simulink model "v2021_10_27_Modello_SITL_AENEA_2020b"  (R2020b)
settings: Solver=ode4  StartTime=0.0  StopTime=0.01  FixedStep=0.01  RelTol=1e-3
values from neighbouring files (symbols this model uses):
  alphavec_rad = deg2rad(alphavec)    [v2021_10_27_calcoloAerodinamica.m]
  attuatore_Amax = 20*(pi/180)    (= 0.349065850399)    [v2021_10_27_avvioSITL.m]    (also in v2021_10_27_calcoloAerodinamica.m)
  attuatore_Emax = 25*(pi/180)    (= 0.436332312999)    [v2021_10_27_avvioSITL.m]    (also in v2021_10_27_calcoloAerodinamica.m)
  attuatore_Rmax = 25*(pi/180)    (= 0.436332312999)    [v2021_10_27_avvioSITL.m]    (also in v2021_10_27_calcoloAerodinamica.m)
  b = 2.62    [v2021_10_27_calcoloAerodinamica.m]
  betavec_rad = deg2rad(betavec)    [v2021_10_27_calcoloAerodinamica.m]
  c = .32    (= 0.32)    [v2021_10_27_calcoloAerodinamica.m]
  cbar = .32    (= 0.32)    [v2021_10_27_calcoloAerodinamica.m]
  CD0 = 0.024    [v2021_10_27_calcoloAerodinamica.m]
  Clp = -0.5058    [v2021_10_27_calcoloAerodinamica.m]
  CLq = 19.166    [v2021_10_27_calcoloAerodinamica.m]
  Clr = 0.1459    [v2021_10_27_calcoloAerodinamica.m]
  Cmq = -81.796    [v2021_10_27_calcoloAerodinamica.m]
  Cnp = 0.007507    [v2021_10_27_calcoloAerodinamica.m]
  Cnr = -1.2593    [v2021_10_27_calcoloAerodinamica.m]
  CYp = 0.050728    [v2021_10_27_calcoloAerodinamica.m]
  CYr = 0.358925    [v2021_10_27_calcoloAerodinamica.m]
  deltaAtrim = 0    [v2021_10_27_avvioSITL.m]
  deltaEtrim = 0    [v2021_10_27_avvioSITL.m]
  deltaRtrim = 0    [v2021_10_27_avvioSITL.m]
  deltaTtrim = 0.1    [v2021_10_27_avvioSITL.m]
  Dprop = 2*Rprop    (= 0.5334)    [v2021_10_27_calcoloAerodinamica.m]
  g = [0 0 9.81]'    [v2021_10_27_calcoloAerodinamica.m]
  HINI = -State0.Pos0(3)    [v2021_10_27_avvioSITL.m]
  Jeng = 0    [v2021_10_27_calcoloAerodinamica.m]
  Jprop = mprop*(Dprop^2)/12    (= 0.00422031414)    [v2021_10_27_calcoloAerodinamica.m]
  latitudineINI = 41.854432*pi/180    (= 0.730497644952)    [v2021_10_27_avvioSITL.m]
  longitudineINI = 12.306650*pi/180    (= 0.214791562391)    [v2021_10_27_avvioSITL.m]
  matricepolinomi = [0.0816560564319 0.0869820125665 0.0279748858868 -4.51852057237 0.0146653626785 -0.925775006168 8.18052218957e-06 -1.47322908992e-05 7.59644694438e-06 0.00246695371279 9.02269223066e-06 0.000559334242525 ... (126 elements, 6x21)]    [coefficienti_curve_renard.mat]
  PWM_Aileron = rad2deg(deltaAtrim)*9+1503    [v2021_10_27_avvioSITL.m]
  PWM_Elevator = rad2deg(deltaEtrim)*(447/50)+(3007/2)    [v2021_10_27_avvioSITL.m]
  PWM_Rudder = rad2deg(deltaRtrim)*(447/50)+(3007/2)    [v2021_10_27_avvioSITL.m]
  PWM_Throttle = (deltaTtrim)*800+1100    (= 1180)    [v2021_10_27_avvioSITL.m]
  q = stato(11)    [measure_F1B.m]
  r = stato(12)    [measure_F1B.m]
  rACtG = rACtP-rGP    [v2021_10_27_calcoloAerodinamica.m]
  rACwG = rACwP-rGP    [v2021_10_27_calcoloAerodinamica.m]
  rAHRSG = rAHRSP-rGP    [v2021_10_27_calcoloAerodinamica.m]
  rho = 1.21330    (= 1.2133)    [v2021_10_27_calcoloAerodinamica.m]
  rLEG = rLEP-rGP    [v2021_10_27_calcoloAerodinamica.m]
  rmglG = rmglP-rGP    [v2021_10_27_calcoloAerodinamica.m]
  rmgrG = rmgrP-rGP    [v2021_10_27_calcoloAerodinamica.m]
  rngG = rngP-rGP    [v2021_10_27_calcoloAerodinamica.m]
  rNPG = rNPP-rGP    [v2021_10_27_calcoloAerodinamica.m]
  rPG = -rGP    [v2021_10_27_calcoloAerodinamica.m]
  Rprop = 0.2667    [v2021_10_27_calcoloAerodinamica.m]
  S = b*cbar    (= 0.8384)    [v2021_10_27_calcoloAerodinamica.m]
  sensori_FreqCampionamento_pitot = 0.02    [v2021_10_27_avvioSITL.m]
  sensori_RumoreSampleTime = 0.02    [v2021_10_27_avvioSITL.m]
  sensori_varianza = 0.0000    (= 0)    [v2021_10_27_avvioSITL.m]
  tsamp = 0.02    [v2021_10_27_avvioSITL.m]
  V_cruise = input('inserire un valore desiderato per V_cruise: ')    [trimCalc.m]    (also in v2021_10_27_trimCalc.m = input('inserire un valore desiderato per V_cruise [m/s]: '))
  W = m*g    [v2021_10_27_calcoloAerodinamica.m]
  WP_AL = [     0 20 0 0 41.807822 12.589274 3 ... (first row only)    [v2021_10_27_avvioSITL.m]
  WP_db_info = [0 0 0 0 1 3;              0 0 0 0 2 3;              0 0 0 0 3 3;              0 0 0 0 0 0]    [v2021_10_27_avvioSITL.m]
  WP_db_param = [ ... (first row only)    [v2021_10_27_avvioSITL.m]
  Zeng = rPG(3)    [v2021_10_27_calcoloAerodinamica.m]
  Zpista = 0    [v2021_10_27_avvioSITL.m]
undefined symbols (not defined in the file or in its folder): beta_phi, beta_psi, beta_theta, CldA, CLdE, CldR, CmdE, CndA, CndR, CYdA, CYdR, delay_ahrs, delay_bmp, delay_gps, Earth, F, h_home, J_vec, mean_ax, mean_ay, mean_az, mean_p, mean_q, mean_r, MIL, P_ref, Receive, seed_ahrs, seed_baro, seed_gps, Send, State0, Std_con_lat, Std_con_long, Std_vel, T0_ref, Ta_lat, Ta_long, Ts_ahrs, Ts_bmp, Ts_gps, Var_heading_static, Var_V_hor_static, WGS84, White_ax, White_ay, White_az, White_gm_phi, White_gm_psi, White_gm_theta, White_p, White_pressione, White_r
libraries: simulink_extras x27, aerolibfltsims x5, aerolibwind2 x3, aerolibasang x2, simulink x2, shared6dof x1, pid_lib x1, aerolibatmos2 x1, aerolibanimutils x1
(part 2 of 3)

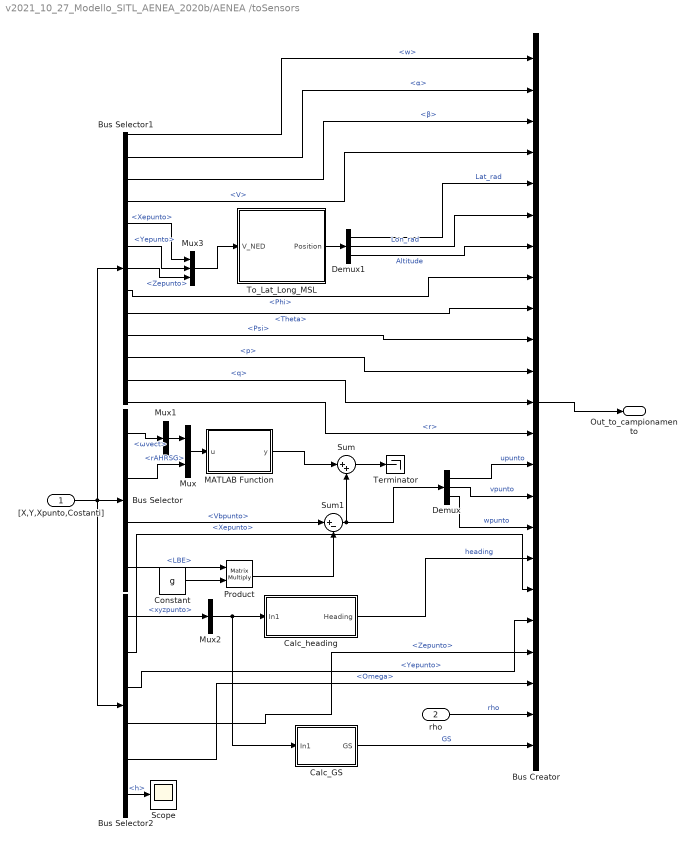
== system v2021_10_27_Modello_SITL_AENEA_2020b/AENEA /toSensors ==
  "[X,Y,Xpunto,Costanti]" : Inport
  rho : Inport  Port=2
  Bus Creator : BusCreator  Inputs=23
  Bus Selector : BusSelector  OutputSignals=X.ωvect,Costanti.Vett_caratteristici.rAHRSG,Xpunto.Vbpunto,Y.LBE
  Bus Selector1 : BusSelector  OutputSignals=X.uvw.w,Y.Vbpolare.α,Y.Vbpolare.β,Y.Vbpolare.V,Xpunto.xyzpunto.Xepunto,Xpunto.xyzpunto.Yepunto,Xpunto.xyzpunto.Zepunto,X.PhiThetaPsi.Phi,X.PhiThetaPsi.Theta,X.PhiThetaPsi.Psi,X.ωvect.p,X.ωvect.q,X.ωvect.r
  Bus Selector2 : BusSelector  OutputSignals=Xpunto.xyzpunto,Xpunto.xyzpunto.Xepunto,Xpunto.xyzpunto.Yepunto,Xpunto.xyzpunto.Zepunto,Y.Omega,X.xyz.h
  Calc_GS : Subsystem
  Calc_heading : Subsystem
  Constant : Constant  Value=g
  Demux : Demux  Outputs=3
  Demux1 : Demux  Outputs=3
  MATLAB Function : MATLAB Function  TreatAsAtomicUnit=on
  Mux : Mux  Inputs=2
  Mux1 : Mux  Inputs=1
  Mux2 : Mux  Inputs=1
  Mux3 : Mux  Inputs=3
  Product : Product  Multiplication=Matrix(*)
  Scope : Scope
  Sum : Sum  Inputs=|++
  Sum1 : Sum  Inputs=|+-
  Terminator : Terminator
  To_Lat_Long_MSL : Subsystem
  Out_to_campionamento : Outport  VectorParamsAs1DForOutWhenUnconnected=off
  wires:
  "[X,Y,Xpunto,Costanti]"/1 -> Bus Selector2/1, Bus Selector1/1, Bus Selector/1
  Mux/1 -> MATLAB Function/1(u)
  Mux1/1 -> Mux/1
  Bus Selector/4 -> Product/1  "<LBE>"
  Constant/1 -> Product/2
  Mux2/1 -> Calc_GS/1(In1), Calc_heading/1(In1)
  Bus Selector2/1 -> Mux2/1  "<xyzpunto>"
  Bus Selector1/1 -> Bus Creator/1  "<w>"
  Bus Selector1/2 -> Bus Creator/2  "<α>"
  Bus Selector1/3 -> Bus Creator/3  "<β>"
  Bus Creator/1 -> Out_to_campionamento/1
  Bus Selector1/4 -> Bus Creator/4  "<V>"
  Bus Selector1/8 -> Bus Creator/8  "<Phi>"
  Bus Selector1/9 -> Bus Creator/9  "<Theta>"
  Bus Selector1/10 -> Bus Creator/10  "<Psi>"
  Bus Selector1/11 -> Bus Creator/11  "<p>"
  Bus Selector1/12 -> Bus Creator/12  "<q>"
  Bus Selector1/13 -> Bus Creator/13  "<r>"
  Demux/1 -> Bus Creator/14  "upunto"
  Demux/2 -> Bus Creator/15  "vpunto"
  Demux/3 -> Bus Creator/16  "wpunto"
  Calc_heading/1(Heading) -> Bus Creator/17  "heading"
  Bus Selector2/5 -> Bus Creator/21  "<Omega>"
  rho/1 -> Bus Creator/22  "rho"
  Calc_GS/1(GS) -> Bus Creator/23  "GS"
  Mux3/1 -> To_Lat_Long_MSL/1(V_NED)
  Bus Selector1/7 -> Mux3/3  "<Zepunto>"
  Bus Selector1/6 -> Mux3/2  "<Yepunto>"
  Bus Selector1/5 -> Mux3/1  "<Xepunto>"
  To_Lat_Long_MSL/1(Position) -> Demux1/1
  Demux1/1 -> Bus Creator/5  "Lat_rad"
  Demux1/2 -> Bus Creator/6  "Lon_rad"
  Demux1/3 -> Bus Creator/7  "Altitude"
  Bus Selector2/2 -> Bus Creator/18  "<Xepunto>"
  Bus Selector2/3 -> Bus Creator/19  "<Yepunto>"
  Bus Selector2/4 -> Bus Creator/20  "<Zepunto>"
  Bus Selector/1 -> Mux1/1  "<ωvect>"
  Bus Selector/2 -> Mux/2  "<rAHRSG>"
  MATLAB Function/1(y) -> Sum/1
  Sum/1 -> Terminator/1
  Product/1 -> Sum1/2
  Bus Selector2/6 -> Scope/1  "<h>"
  Sum1/1 -> Demux/1, Sum/2
  Bus Selector/3 -> Sum1/1  "<Vbpunto>"

== system v2021_10_27_Modello_SITL_AENEA_2020b/Ricezione segnali2/Subsystem1 ==
  In1 : Inport
  In2 : Inport  Port=2
  In3 : Inport  Port=3
  In4 : Inport  Port=4
  AILERON : Subsystem
  Degrees to Radians : simulink_extras/Transformations/Degrees to Radians
  Degrees to Radians1 : simulink_extras/Transformations/Degrees to Radians
  Degrees to Radians2 : simulink_extras/Transformations/Degrees to Radians
  ELEVATOR : Subsystem
  RUDDER : Subsystem
  Scope : Scope  NumInputPorts=2
  Scope1 : Scope
  Scope2 : Scope  NumInputPorts=2
  Scope3 : Scope
  Scope4 : Scope
  THROTTLE : Subsystem
  Out1 : Outport  VectorParamsAs1DForOutWhenUnconnected=off
  Out2 : Outport  Port=2  VectorParamsAs1DForOutWhenUnconnected=off
  Out3 : Outport  Port=3  VectorParamsAs1DForOutWhenUnconnected=off
  Out4 : Outport  Port=4  VectorParamsAs1DForOutWhenUnconnected=off
  wires:
  In3/1 -> AILERON/1(In1)
  In4/1 -> RUDDER/1(In1)
  In2/1 -> Scope/1, ELEVATOR/1(In1)
  In1/1 -> Scope2/1, THROTTLE/1(In1)
  Degrees to Radians2/1 -> Out4/1, Scope4/1  "Timone"
  Degrees to Radians1/1 -> Out3/1, Scope3/1  "Alettoni"
  Degrees to Radians/1 -> Scope/2, Scope1/1, Out2/1  "Equilibratore"
  THROTTLE/1(Out1) -> Scope2/2, Out1/1  "Manetta"
  ELEVATOR/1(Out1) -> Degrees to Radians/1  "Equilibratore"
  AILERON/1(Out1) -> Degrees to Radians1/1  "Alettoni"
  RUDDER/1(Out1) -> Degrees to Radians2/1  "Timone"

== system v2021_10_27_Modello_SITL_AENEA_2020b/ 1/GPS1/Subsystem ==
  Lat : Inport
  C/Lat1 : Constant  Value=Std_con_lat
  Delay_gps : TransportDelay  DelayTime=delay_gps  InitialOutput=latitudineINI
  Gain : Gain  Gain=1/Ta_lat  SaturateOnIntegerOverflow=on  OutDataTypeStr=Inherit: Same as input  ParamDataTypeStr=Inherit: Same as input
  Integrator : Integrator
  Multiply : Product
  Multiply1 : Product
  Sum : Sum  Inputs=|+-  InputSameDT=on  SaturateOnIntegerOverflow=on  OutDataTypeStr=Inherit: Same as first input
  Sum1 : Sum  Inputs=|++  InputSameDT=on  SaturateOnIntegerOverflow=on  OutDataTypeStr=Inherit: Same as first input
  To Workspace : ToWorkspace  Commented=on  VariableName=errore_lat  SaveFormat=Timeseries  SampleTime=-1
  White Noise : RandomNumber  Seed=seed_gps  SampleTime=Ts_gps
  Out1 : Outport  VectorParamsAs1DForOutWhenUnconnected=off
  wires:
  Sum1/1 -> Out1/1
  Integrator/1 -> Gain/1, Sum1/2, To Workspace/1
  Sum/1 -> Integrator/1
  Delay_gps/1 -> Multiply1/1, Sum1/1
  Gain/1 -> Sum/2
  White Noise/1 -> Multiply/2
  Multiply/1 -> Sum/1
  Lat/1 -> Delay_gps/1
  C/Lat1/1 -> Multiply1/2
  Multiply1/1 -> Multiply/1

== system v2021_10_27_Modello_SITL_AENEA_2020b/ 1/GPS1/Subsystem1 ==
  Long : Inport
  C/Long1 : Constant  Value=Std_con_long
  Delay_gps : TransportDelay  DelayTime=delay_gps  InitialOutput=longitudineINI
  Gain1 : Gain  Gain=1/Ta_long  SaturateOnIntegerOverflow=on  OutDataTypeStr=Inherit: Same as input  ParamDataTypeStr=Inherit: Same as input
  Integrator : Integrator
  Multiply : Product
  Multiply1 : Product
  Sum : Sum  Inputs=|+-  InputSameDT=on  SaturateOnIntegerOverflow=on  OutDataTypeStr=Inherit: Same as first input
  Sum1 : Sum  Inputs=|++  InputSameDT=on  SaturateOnIntegerOverflow=on  OutDataTypeStr=Inherit: Same as first input
  To Workspace : ToWorkspace  VariableName=errore_long  SaveFormat=Timeseries  SampleTime=-1
  White Noise : RandomNumber  Seed=seed_gps  SampleTime=Ts_gps
  long_out : Outport  VectorParamsAs1DForOutWhenUnconnected=off
  wires:
  Multiply/1 -> Sum/1
  White Noise/1 -> Multiply/2
  Gain1/1 -> Sum/2
  Sum1/1 -> long_out/1
  Delay_gps/1 -> Multiply1/1, Sum1/1
  Sum/1 -> Integrator/1
  Integrator/1 -> Sum1/2, To Workspace/1, Gain1/1
  Multiply1/1 -> Multiply/1
  C/Long1/1 -> Multiply1/2
  Long/1 -> Delay_gps/1

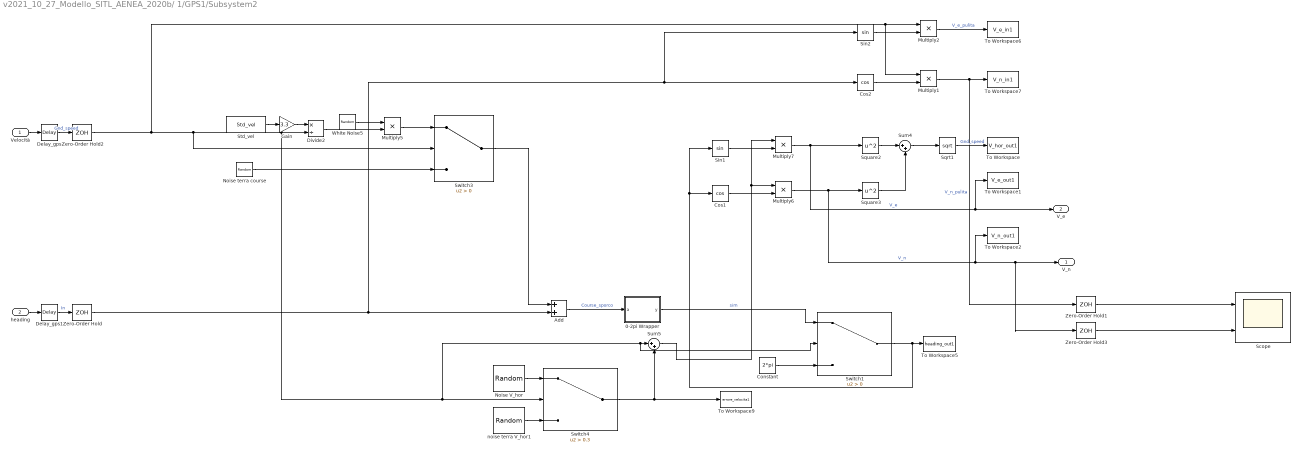
== system v2021_10_27_Modello_SITL_AENEA_2020b/ 1/GPS1/Subsystem2 ==
  Velocità : Inport
  heading : Inport  Port=2
  0-2pi Wrapper : MATLAB Function  TreatAsAtomicUnit=on
  Add : Sum
  Constant : Constant  Value=2*pi
  Cos1 : Trigonometry  Operator=cos
  Cos2 : Trigonometry  Operator=cos
  Delay_gps : TransportDelay  DelayTime=delay_gps  InitialOutput=V_cruise
  Delay_gps1 : TransportDelay  DelayTime=delay_gps
  Divide2 : Product  Inputs=*/
  Gain : Gain  Gain=3.3
  Multiply{1..2,5..7} (5 alike) : Product
  Noise V_hor : RandomNumber  Variance=Std_vel^2  Seed=seed_gps  SampleTime=Ts_gps
  Noise terra course : RandomNumber  Variance=Var_heading_static  Seed=seed_gps  SampleTime=0.02
  Scope : Scope  NumInputPorts=2
  Sin1 : Trigonometry
  Sin2 : Trigonometry
  Sqrt1 : Sqrt  SaturateOnIntegerOverflow=on
  Square2 : Math  Operator=square  SignedPower=on  SaturateOnIntegerOverflow=on
  Square3 : Math  Operator=square  SignedPower=on  SaturateOnIntegerOverflow=on
  Std_vel : Constant  Value=Std_vel
  Sum4 : Sum  Inputs=|++
  Sum5 : Sum  Inputs=|++
  Switch1 : Switch  Criteria=u2 > Threshold
  Switch3 : Switch  Criteria=u2 > Threshold
  Switch4 : Switch  Criteria=u2 > Threshold  Threshold=0.3
  To Workspace : ToWorkspace  VariableName=V_hor_out1  SaveFormat=Timeseries  SampleTime=-1
  To Workspace1 : ToWorkspace  VariableName=V_e_out1  SaveFormat=Timeseries  SampleTime=-1
  To Workspace2 : ToWorkspace  VariableName=V_n_out1  SaveFormat=Timeseries  SampleTime=-1
  To Workspace5 : ToWorkspace  VariableName=heading_out1  SaveFormat=Timeseries  SampleTime=-1
  To Workspace6 : ToWorkspace  VariableName=V_e_in1  SaveFormat=Timeseries  SampleTime=-1
  To Workspace7 : ToWorkspace  VariableName=V_n_in1  SaveFormat=Timeseries  SampleTime=-1
  To Workspace9 : ToWorkspace  VariableName=errore_velocita1  SaveFormat=Timeseries  SampleTime=-1
  White Noise5 : RandomNumber  Variance=0.1  Seed=seed_gps  SampleTime=0.02
  Zero-Order Hold : ZeroOrderHold  SampleTime=0.02
  Zero-Order Hold1 : ZeroOrderHold  SampleTime=0.2
  Zero-Order Hold2 : ZeroOrderHold  SampleTime=0.02
  Zero-Order Hold3 : ZeroOrderHold  SampleTime=0.2
  noise terra V_hor1 : RandomNumber  Variance=Var_V_hor_static  Seed=seed_gps  SampleTime=Ts_gps
  "V_n " : Outport  VectorParamsAs1DForOutWhenUnconnected=off
  V_e : Outport  Port=2  VectorParamsAs1DForOutWhenUnconnected=off
  wires:
  Zero-Order Hold2/1 -> Multiply2/1, Multiply1/1, Switch3/2, Divide2/2, Switch4/2, Sum5/1, Switch1/2
  Zero-Order Hold/1 -> Add/2, Sin2/1, Cos2/1
  Switch1/1 -> To Workspace5/1, Cos1/1, Sin1/1
  Constant/1 -> Switch1/3
  Sqrt1/1 -> To Workspace/1  "Gnd_speed"
  Divide2/1 -> Multiply5/2
  Velocità/1 -> Delay_gps/1
  heading/1 -> Delay_gps1/1
  Sin2/1 -> Multiply2/2
  Sin1/1 -> Multiply7/2
  Noise terra course/1 -> Switch3/3
  0-2pi Wrapper/1(y) -> Switch1/1  "sim"
  Cos2/1 -> Multiply1/2
  Multiply2/1 -> To Workspace6/1  "V_e_pulita"
  Multiply1/1 -> Zero-Order Hold1/1, To Workspace7/1  "V_n_pulita"
  Noise V_hor/1 -> Switch4/1
  Switch3/1 -> Add/1
  Cos1/1 -> Multiply6/2
  Sum4/1 -> Sqrt1/1
  Multiply7/1 -> Square2/1, V_e/1, To Workspace1/1  "V_e"
  White Noise5/1 -> Multiply5/1
  Delay_gps/1 -> Zero-Order Hold2/1  "Gnd_speed"
  Sum5/1 -> Multiply7/1, Multiply6/1
  Multiply6/1 -> Square3/1, To Workspace2/1, Zero-Order Hold3/1, "V_n "/1  "V_n"
  Square2/1 -> Sum4/1
  Multiply5/1 -> Switch3/1
  Add/1 -> 0-2pi Wrapper/1(a)  "Course_sporco"
  Delay_gps1/1 -> Zero-Order Hold/1  "In"
  Square3/1 -> Sum4/2
  noise terra V_hor1/1 -> Switch4/3
  Switch4/1 -> Sum5/2, To Workspace9/1
  Zero-Order Hold1/1 -> Scope/1
  Zero-Order Hold3/1 -> Scope/2
  Std_vel/1 -> Gain/1
  Gain/1 -> Divide2/1

== system v2021_10_27_Modello_SITL_AENEA_2020b/ 1/int1/INT16  ==
  <u> : Inport
  Data Type Conversion : DataTypeConversion  OutDataTypeStr=int16  LockScale=on
  Data Type Conversion1 : DataTypeConversion  OutDataTypeStr=double  LockScale=on
  Gain : Gain  Gain=100
  Gain1 : Gain  Gain=1/100
  Out1 : Outport  VectorParamsAs1DForOutWhenUnconnected=off
  wires:
  <u>/1 -> Gain/1
  Gain1/1 -> Out1/1
  Gain/1 -> Data Type Conversion/1
  Data Type Conversion/1 -> Data Type Conversion1/1
  Data Type Conversion1/1 -> Gain1/1

== system v2021_10_27_Modello_SITL_AENEA_2020b/ 1/int16/INT16  ==
  <u> : Inport
  Data Type Conversion : DataTypeConversion  OutDataTypeStr=int16  LockScale=on
  Data Type Conversion1 : DataTypeConversion  OutDataTypeStr=double  LockScale=on
  Gain : Gain  Gain=100
  Gain1 : Gain  Gain=1/100
  Out1 : Outport  VectorParamsAs1DForOutWhenUnconnected=off
  wires:
  Data Type Conversion1/1 -> Gain1/1
  Data Type Conversion/1 -> Data Type Conversion1/1
  Gain/1 -> Data Type Conversion/1
  Gain1/1 -> Out1/1
  <u>/1 -> Gain/1

== system v2021_10_27_Modello_SITL_AENEA_2020b/ 1/int16_rad /INT16  ==
  <u> : Inport
  Data Type Conversion : DataTypeConversion  OutDataTypeStr=int16  LockScale=on
  Data Type Conversion1 : DataTypeConversion  OutDataTypeStr=double  LockScale=on
  Gain : Gain  Gain=100
  Gain1 : Gain  Gain=1/100
  Out1 : Outport  VectorParamsAs1DForOutWhenUnconnected=off
  wires:
  <u>/1 -> Gain/1
  Gain1/1 -> Out1/1
  Gain/1 -> Data Type Conversion/1
  Data Type Conversion/1 -> Data Type Conversion1/1
  Data Type Conversion1/1 -> Gain1/1

== system v2021_10_27_Modello_SITL_AENEA_2020b/ 1/int16_rad 1/INT16  ==
  <u> : Inport
  Data Type Conversion : DataTypeConversion  OutDataTypeStr=int16  LockScale=on
  Data Type Conversion1 : DataTypeConversion  OutDataTypeStr=double  LockScale=on
  Gain : Gain  Gain=100
  Gain1 : Gain  Gain=1/100
  Out1 : Outport  VectorParamsAs1DForOutWhenUnconnected=off
  wires:
  Data Type Conversion1/1 -> Gain1/1
  Data Type Conversion/1 -> Data Type Conversion1/1
  Gain/1 -> Data Type Conversion/1
  Gain1/1 -> Out1/1
  <u>/1 -> Gain/1

== system v2021_10_27_Modello_SITL_AENEA_2020b/ 1/int16_rad 2/INT16  ==
  <u> : Inport
  Data Type Conversion : DataTypeConversion  OutDataTypeStr=int16  LockScale=on
  Data Type Conversion1 : DataTypeConversion  OutDataTypeStr=double  LockScale=on
  Gain : Gain  Gain=100
  Gain1 : Gain  Gain=1/100
  Out1 : Outport  VectorParamsAs1DForOutWhenUnconnected=off
  wires:
  <u>/1 -> Gain/1
  Gain1/1 -> Out1/1
  Gain/1 -> Data Type Conversion/1
  Data Type Conversion/1 -> Data Type Conversion1/1
  Data Type Conversion1/1 -> Gain1/1

== system v2021_10_27_Modello_SITL_AENEA_2020b/ 1/int16_rad 3/INT16  ==
  <u> : Inport
  Data Type Conversion : DataTypeConversion  OutDataTypeStr=int16  LockScale=on
  Data Type Conversion1 : DataTypeConversion  OutDataTypeStr=double  LockScale=on
  Gain : Gain  Gain=100
  Gain1 : Gain  Gain=1/100
  Out1 : Outport  VectorParamsAs1DForOutWhenUnconnected=off
  wires:
  Data Type Conversion1/1 -> Gain1/1
  Data Type Conversion/1 -> Data Type Conversion1/1
  Gain/1 -> Data Type Conversion/1
  Gain1/1 -> Out1/1
  <u>/1 -> Gain/1

== system v2021_10_27_Modello_SITL_AENEA_2020b/ 1/int16_rad 4/INT16  ==
  <u> : Inport
  Data Type Conversion : DataTypeConversion  OutDataTypeStr=int16  LockScale=on
  Data Type Conversion1 : DataTypeConversion  OutDataTypeStr=double  LockScale=on
  Gain : Gain  Gain=100
  Gain1 : Gain  Gain=1/100
  Out1 : Outport  VectorParamsAs1DForOutWhenUnconnected=off
  wires:
  <u>/1 -> Gain/1
  Gain1/1 -> Out1/1
  Gain/1 -> Data Type Conversion/1
  Data Type Conversion/1 -> Data Type Conversion1/1
  Data Type Conversion1/1 -> Gain1/1

== system v2021_10_27_Modello_SITL_AENEA_2020b/ 1/int16_rad 5/INT16  ==
  <u> : Inport
  Data Type Conversion : DataTypeConversion  OutDataTypeStr=int16  LockScale=on
  Data Type Conversion1 : DataTypeConversion  OutDataTypeStr=double  LockScale=on
  Gain : Gain  Gain=100
  Gain1 : Gain  Gain=1/100
  Out1 : Outport  VectorParamsAs1DForOutWhenUnconnected=off
  wires:
  Data Type Conversion1/1 -> Gain1/1
  Data Type Conversion/1 -> Data Type Conversion1/1
  Gain/1 -> Data Type Conversion/1
  Gain1/1 -> Out1/1
  <u>/1 -> Gain/1

== system v2021_10_27_Modello_SITL_AENEA_2020b/ 1/int2/INT16  ==
  <u> : Inport
  Data Type Conversion : DataTypeConversion  OutDataTypeStr=int16  LockScale=on
  Data Type Conversion1 : DataTypeConversion  OutDataTypeStr=double  LockScale=on
  Gain : Gain  Gain=100
  Gain1 : Gain  Gain=1/100
  Out1 : Outport  VectorParamsAs1DForOutWhenUnconnected=off
  wires:
  Data Type Conversion1/1 -> Gain1/1
  Data Type Conversion/1 -> Data Type Conversion1/1
  Gain/1 -> Data Type Conversion/1
  Gain1/1 -> Out1/1
  <u>/1 -> Gain/1

== system v2021_10_27_Modello_SITL_AENEA_2020b/AENEA /AENEA II_SITL1/Forze aerodinamiche ==
  ωb : Inport
  qbar : Inport  Port=2
  Vect_Comandi : Inport  Port=3
  Vect_Costanti : Inport  Port=4
  "Vbpolare " : Inport  Port=5
  Bus Creator : BusCreator  Inputs=3
  Bus Selector : BusSelector  OutputSignals=α,β
  Bus Selector1 : BusSelector  OutputSignals=Coef_Geometrici.S
  Demux : Demux  Outputs=3
  Forze assi vento/q : Subsystem
  MATLAB Function : MATLAB Function  TreatAsAtomicUnit=on
  Matrix Multiply : Product  Multiplication=Matrix(*)
  Momenti /press din : Subsystem
  Product : Product  Inputs=3
  Product2 : Product
  FA_B : Outport  VectorParamsAs1DForOutWhenUnconnected=off
  MA_B : Outport  Port=2  VectorParamsAs1DForOutWhenUnconnected=off
  CL : Outport  Port=3  VectorParamsAs1DForOutWhenUnconnected=off
  wires:
  Product2/1 -> MA_B/1
  Product/1 -> FA_B/1
  qbar/1 -> Product/3, Product2/1
  ωb/1 -> Demux/1
  Demux/1 -> Bus Creator/1  "p"
  Demux/2 -> Bus Creator/2  "q"
  Demux/3 -> Bus Creator/3  "r"
  Bus Selector/1 -> MATLAB Function/1(alpha)  "<α>"
  Bus Selector/2 -> MATLAB Function/2(beta)  "<β>"
  MATLAB Function/1(Lbw) -> Matrix Multiply/1
  Matrix Multiply/1 -> Product/2  "FA_B/q"
  Momenti /press din/1(MA_B/q) -> Product2/2
  Forze assi vento/q/1(FA_W/q) -> Matrix Multiply/2
  Vect_Comandi/1 -> Forze assi vento/q/1(Vect_Comandi), Momenti /press din/1(Vect_Comandi)
  "Vbpolare "/1 -> Bus Selector/1, Forze assi vento/q/3("Vbpolare "), Momenti /press din/3("Vbpolare ")
  Bus Creator/1 -> Momenti /press din/4(ωb), Forze assi vento/q/4(ωb)  "ωb"
  Vect_Costanti/1 -> Bus Selector1/1, Forze assi vento/q/2(Vect_Costanti), Momenti /press din/2(Vect_Costanti)
  Bus Selector1/1 -> Product/1  "<S>"
  Forze assi vento/q/2(CL) -> CL/1

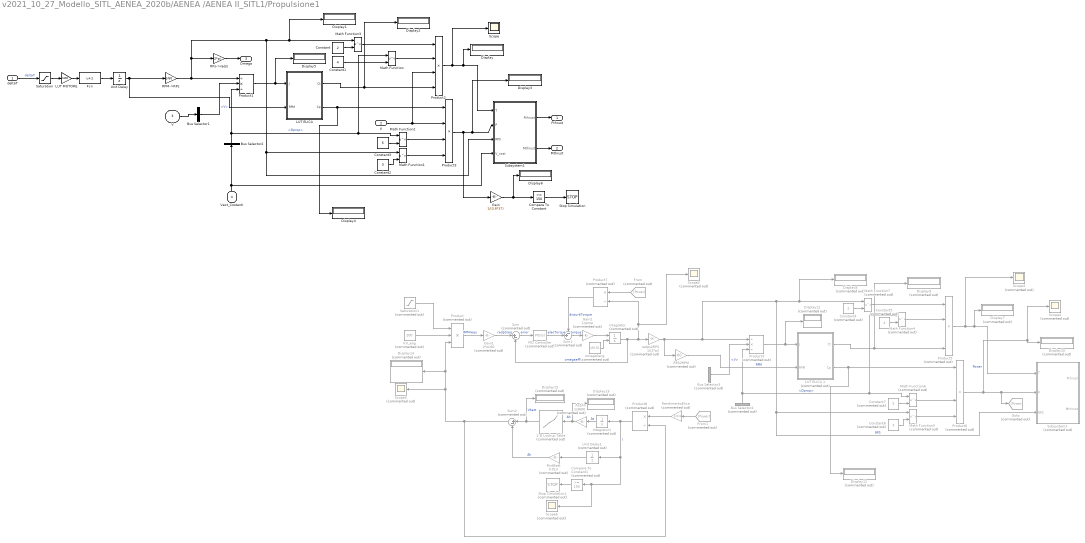
== system v2021_10_27_Modello_SITL_AENEA_2020b/AENEA /AENEA II_SITL1/Propulsione1 ==
  "deltaT " : Inport
  ρ : Inport  Port=2
  V : Inport  Port=3
  Vect_Costanti : Inport  Port=4
  1-D Lookup Table : Lookup_n-D  Commented=on  NumberOfTableDimensions=1  BreakpointsForDimension1=[0,5,5.2]  Table=[42,34,0]  InternalRulePriority=Speed  RndMeth=Simplest  InputSameDT=on
  As2Ah : Gain  Commented=on  Gain=1/3600
  Bus Selector1 : BusSelector  OutputSignals=V
  Bus Selector2 : BusSelector  OutputSignals=Coef_Geometrici.Dprop
  Bus Selector3 : BusSelector  Commented=on  OutputSignals=V
  Bus Selector4 : BusSelector  Commented=on  OutputSignals=Coef_Geometrici.Dprop
  Compare To Constant : simulink/Logic and Bit Operations/Compare To Constant  relop=>=  const=150  OutDataTypeStr=boolean
  Compare To Constant1 : simulink/Logic and Bit Operations/Compare To Constant  Commented=on  relop=>=  const=150  OutDataTypeStr=boolean
  Constant : Constant  Value=2
  Constant1 : Constant  Value=4
  Constant2 : Constant  Value=3
  Constant3 : Constant  Value=5
  Constant4 : Constant  Commented=on  Value=2
  Constant5 : Constant  Commented=on  Value=4
  Constant6 : Constant  Commented=on  Value=3
  Constant7 : Constant  Commented=on  Value=5
  Display{,1..6} (7 alike) : Display
  Display{7..15} (9 alike) : Display  Commented=on
  Fcn : Fcn  Expr=u+1
  From : From  Commented=on  GotoTag=Power
  From1 : From  Commented=on  GotoTag=Power
  Gain : Gain  Gain=1/(0.8*37)
  Gain1 : Gain  Commented=on  Gain=2*pi/60
  Gain2 : Gain  Commented=on  Gain=1/Jprop
  Goto : Goto  Commented=on  GotoTag=Power
  Integrator : Integrator  Commented=on  InitialConditionSource=external
  Integrator1 : Integrator  Commented=on
  "KV_eng " : Constant  Commented=on  Value=200
  "LUT ELICA " : Subsystem
  LUT ELICA 1 : Subsystem  Commented=on
  LUT MOTORE : Gain  Gain=7400
  Math Function{,1..3} (4 alike) : Math  Operator=pow  SignedPower=on  SaturateOnIntegerOverflow=on
  Math Function{4..7} (4 alike) : Math  Commented=on  Operator=pow  SignedPower=on  SaturateOnIntegerOverflow=on
  PID Controller : pid_lib/PID Controller  Commented=on  Controller=PID  Form=Parallel  TimeDomain=Continuous-time  UseExternalTs=off  SampleTime=-1  IntegratorMethod=Forward Euler  FilterMethod=Forward Euler  ControllerParametersSource=internal  P=0.7  I=0.1  D=0  UseFilter=on  N=100  TunerSelectOption=Frequency Response Based  InitialConditionSource=internal  InitialConditionForIntegrator=0  InitialConditionForFilter=0  DifferentiatorICPrevScaledInput=0  ExternalReset=none  TrackingMode=off  Kt=1  LimitOutput=off  SatLimitsSource=internal  UpperSaturationLimit=inf  LowerSaturationLimit=-inf  LinearizeAsGain=on  AntiWindupMode=none  Kb=1  POutMin=[]  POutMax=[]  IOutMin=[]  IOutMax=[]  DOutMin=[]  DOutMax=[]  NOutMin=[]  NOutMax=[]  SumOutMin=[]  SumOutMax=[]  SaturationOutMin=[]  SaturationOutMax=[]  PParamMin=[]  PParamMax=[]  IParamMin=[]  IParamMax=[]  DParamMin=[]  DParamMax=[]  NParamMin=[]  NParamMax=[]  KbParamMin=[]  KbParamMax=[]  KtParamMin=[]  KtParamMax=[]  KbOutMin=[]  KbOutMax=[]  KtOutMin=[]  KtOutMax=[]  IntegratorOutMin=[]  IntegratorOutMax=[]  FilterOutMin=[]  FilterOutMax=[]  SumI1OutMin=[]  SumI1OutMax=[]  SumI2OutMin=[]  SumI2OutMax=[]  SumI3OutMin=[]  SumI3OutMax=[]  SumI4OutMin=[]  SumI4OutMax=[]  SumDOutMin=[]  SumDOutMax=[]  DifferentiatorOutMin=[]  DifferentiatorOutMax=[]  FilterDiffOutCoefMin=[]  FilterDiffOutCoefMax=[]  ReciprocalOutMin=[]  ReciprocalOutMax=[]  SumDenOutMin=[]  SumDenOutMax=[]  SumNumOutMin=[]  SumNumOutMax=[]  DivideOutMin=[]  DivideOutMax=[]  UdiffTsProdOutMin=[]  UdiffTsProdOutMax=[]  NTsProdOutMin=[]  NTsProdOutMax=[]  UintegralTsProdOutMin=[]  UintegralTsProdOutMax=[]  UngainTsProdOutMin=[]  UngainTsProdOutMax=[]  IntegratorContinuousStateAttributes=''  IntegratorStateMustResolveToSignalObject=off  IntegratorRTWStateStorageClass=Auto  FilterContinuousStateAttributes=''  FilterStateMustResolveToSignalObject=off  FilterRTWStateStorageClass=Auto  ParallelPVariant=InternalParameters  IdealPVariant=Disabled  IVariant=InternalParameters  DVariant=InternalParameters  IntegratorVariant=Continuous  SatVariant=Disabled  AWVariant=Passthrough  PCopyVariant=Disabled  TRVariant=Disabled  FdbkBlocksVariant=Forward  IdealPFdbkVariant=Disabled  SatFdbkVariant=Disabled  DerivativeFilterVariant=ContFilter  NVariant=InternalParameters  NCopyVariant=Disabled  FilterICVariant=InternalICsFilter  IntegratorICVariant=InternalICs  ExternalResetVariant=Disabled  TRSumVariant=Passthrough  SumFdbkVariant=Disabled  SumVariant=Sum_PID  TsampFilterVariant=InternalTs  TsampNgainVariant=Passthrough  TsampIntegralVariant=Passthrough  ExternalSaturationOutDataTypeStr=Inherit: Same as second input
  Product : Product  Commented=on  Inputs=3
  Product1 : Product  Inputs=/*/
  Product2 : Product  Inputs=****
  Product3 : Product  Inputs=****
  Product4 : Product  Commented=on  Inputs=/*/
  Product5 : Product  Commented=on  Inputs=****
  Product6 : Product  Commented=on  Inputs=****
  Product7 : Product  Commented=on  Inputs=*/
  Product8 : Product  Commented=on  Inputs=*/
  RPM->RPs : Gain  Gain=1/60
  "RPS2RPM  " : Gain  Commented=on  Gain=60
  RPs->rad/s : Gain  Gain=2*pi
  "RendimentoElica " : Gain  Commented=on  Gain=1/0.8
  "RintBatt " : Gain  Commented=on  Gain=0.013
  Saturation : Saturate  UpperLimit=1  LowerLimit=0
  Saturation1 : Saturate  Commented=on  UpperLimit=1  LowerLimit=0
  Scope : Scope
  Scope{2..6} (5 alike) : Scope  Commented=on
  Stop Simulation : Stop
  Stop Simulation1 : Stop  Commented=on
  Subsystem1 : Subsystem
  Subsystem2 : Subsystem  Commented=on
  Sum : Sum  Commented=on  Inputs=|+-
  Sum1 : Sum  Commented=on  Inputs=-+|
  Sum2 : Sum  Commented=on  Inputs=|+-
  Unit Delay : UnitDelay  InitialCondition=deltaTtrim*7400  SampleTime=-1  HasFrameUpgradeWarning=on
  Unit Delay1 : UnitDelay  Commented=on  SampleTime=0.01  HasFrameUpgradeWarning=on
  omega0eng : Constant  Commented=on  Value=439.82
  radps2RPS : Gain  Commented=on  Gain=1/(2*pi)
  "Fthrust " : Outport  VectorParamsAs1DForOutWhenUnconnected=off
  Mthrust : Outport  Port=2  VectorParamsAs1DForOutWhenUnconnected=off
  Omega : Outport  Port=3
  wires:
  Vect_Costanti/1 -> Subsystem1/4(V_cost), Bus Selector2/1
  "deltaT "/1 -> Saturation/1  "deltaT"
  V/1 -> Bus Selector1/1
  Bus Selector1/1 -> Product1/2  "<V>"
  Bus Selector2/1 -> Math Function2/1, Math Function/1, Product1/3  "<Dprop>"
  Product1/1 -> "LUT ELICA "/1(J), Display5/1
  ρ/1 -> Product2/3, Product3/2
  "LUT ELICA "/2(Cp) -> Display4/1, Product3/1
  "LUT ELICA "/1(Ct) -> Display2/1, Product2/4
  Math Function3/1 -> Product2/1
  Math Function/1 -> Product2/2
  Constant/1 -> Math Function3/2
  Constant1/1 -> Math Function/2
  Math Function2/1 -> Product3/3
  Constant3/1 -> Math Function2/2
  Constant2/1 -> Math Function1/2
  Math Function1/1 -> Product3/4
  Product2/1 -> Scope/1, Display/1, Subsystem1/1(T)
  Subsystem1/1(Fthrust) -> "Fthrust "/1
  Subsystem1/2("Mthrust ") -> Mthrust/1
  Product3/1 -> Gain/1, Display3/1, Subsystem1/2(P)
  Gain/1 -> Display6/1, Compare To Constant/1
  Compare To Constant/1 -> Stop Simulation/1
  RPs->rad/s/1 -> Omega/1
  RPM->RPs/1 -> RPs->rad/s/1, Subsystem1/3(RPS), Math Function1/1, Display1/1, Math Function3/1, Product1/1
  Saturation/1 -> LUT MOTORE/1
  Unit Delay/1 -> "LUT ELICA "/2(RPM), RPM->RPs/1
  LUT MOTORE/1 -> Fcn/1
  Fcn/1 -> Unit Delay/1
  omega0eng/1 -> Integrator/2
  Saturation1/1 -> Product/1
  Product/1 -> Gain1/1  "RPMrequ"
  From1/1 -> "RendimentoElica "/1
  Product7/1 -> Sum1/1  "disturbTorque"
  "RendimentoElica "/1 -> Product8/1
  "RintBatt "/1 -> Sum2/2  "Ah"
  Unit Delay1/1 -> "RintBatt "/1
  Sum2/1 -> Product8/2, Scope5/1, Display14/1, Product/3
  LUT ELICA 1/1(Ct) -> Display9/1, Product5/4
  Product8/1 -> Scope6/1, Compare To Constant1/1, Unit Delay1/1, Integrator1/1  "I"
  Bus Selector4/1 -> Math Function6/1, Math Function4/1, Product4/3  "<Dprop>"
  PID Controller/1 -> Sum1/2  "elecTorque"
  Integrator/1 -> Sum/2, Scope2/1, Product7/2, radps2RPS/1  "omegaeff"
  1-D Lookup Table/1 -> Display15/1, Sum2/1  "Vbatt"
  "KV_eng "/1 -> Product/2
  Math Function6/1 -> Product6/3
  Gain1/1 -> Sum/1  "radpSreq"
  Product6/1 -> Scope4/1, Display10/1, Goto/1, Subsystem2/2(P)  "Power"
  Sum1/1 -> Gain2/1  "torque"
  Compare To Constant1/1 -> Stop Simulation1/1
  LUT ELICA 1/2(Cp) -> Display11/1, Product6/1
  Integrator1/1 -> As2Ah/1  "As"
  Math Function7/1 -> Product5/1
  Sum/1 -> PID Controller/1  "error"
  As2Ah/1 -> Display13/1, 1-D Lookup Table/1  "Ah"
  Product5/1 -> Scope3/1, Display7/1, Subsystem2/1(T)
  Math Function5/1 -> Product6/4
  "RPS2RPM  "/1 -> LUT ELICA 1/2(RPM)  "RPM"
  From/1 -> Product7/1
  Math Function4/1 -> Product5/2
  Constant4/1 -> Math Function7/2
  Constant6/1 -> Math Function5/2
  Constant7/1 -> Math Function6/2
  Product4/1 -> Display12/1, LUT ELICA 1/1(J)
  radps2RPS/1 -> "RPS2RPM  "/1, Subsystem2/3(RPS), Math Function5/1, Display8/1, Math Function7/1, Product4/1  "RPS"
  Gain2/1 -> Integrator/1
  Bus Selector3/1 -> Product4/2  "<V>"
  Constant5/1 -> Math Function4/2

== system v2021_10_27_Modello_SITL_AENEA_2020b/AENEA /AENEA II_SITL1/Subsystem ==
  xE : Inport
  Φvect : Inport  Port=2
  Vb : Inport  Port=3
  ω_b : Inport  Port=4
  Bus Creator1 : BusCreator  Inputs=4
  Bus Creator{3..4,8..9} (4 alike) : BusCreator  Inputs=3
  Demux{1..2,6..7} (4 alike) : Demux  Outputs=3
  Scope : Scope
  "Xstato " : Outport  VectorParamsAs1DForOutWhenUnconnected=off
  wires:
  Demux2/3 -> Bus Creator4/3  "r"
  Bus Creator4/1 -> Bus Creator1/3  "ωvect"
  Φvect/1 -> Demux6/1
  Vb/1 -> Demux7/1
  Bus Creator8/1 -> Bus Creator1/2  "PhiThetaPsi"
  Demux1/3 -> Bus Creator3/3  "h"
  Demux2/2 -> Bus Creator4/2  "q"
  Demux2/1 -> Bus Creator4/1  "p"
  Bus Creator3/1 -> Bus Creator1/4  "xyz"
  ω_b/1 -> Demux2/1
  Demux6/3 -> Scope/1, Bus Creator8/3  "Psi"
  Demux6/1 -> Bus Creator8/1  "Phi"
  Demux1/1 -> Bus Creator3/1  "x"
  Demux7/1 -> Bus Creator9/1  "u"
  Demux7/3 -> Bus Creator9/3  "w"
  Bus Creator9/1 -> Bus Creator1/1  "uvw"
  Demux1/2 -> Bus Creator3/2  "y"
  Demux7/2 -> Bus Creator9/2  "v"
  Demux6/2 -> Bus Creator8/2  "Theta"
  Bus Creator1/1 -> "Xstato "/1  "Xstato"
  xE/1 -> Demux1/1

== system v2021_10_27_Modello_SITL_AENEA_2020b/AENEA /AENEA II_SITL1/Subsystem1 ==
  omegapunto : Inport
  V : Inport  Port=2
  Abb : Inport  Port=3
  "PhiThetaPsipunto " : Inport  Port=4
  Bus Creator{5,7,10..11} (4 alike) : BusCreator  Inputs=3
  Bus Creator6 : BusCreator  Inputs=4
  Demux{3..4,8..9} (4 alike) : Demux  Outputs=3
  Xpunto : Outport  VectorParamsAs1DForOutWhenUnconnected=off
  wires:
  Demux4/3 -> Bus Creator7/3  "wpunto"
  Demux3/1 -> Bus Creator5/1  "ppunto"
  Demux4/2 -> Bus Creator7/2  "vpunto"
  Demux8/2 -> Bus Creator10/2  "Thetapunto"
  Bus Creator10/1 -> Bus Creator6/2  "EulerAnglespunto"
  Demux3/2 -> Bus Creator5/2  "qpunto"
  Demux4/1 -> Bus Creator7/1  "upunto"
  V/1 -> Demux9/1
  Demux8/1 -> Bus Creator10/1  "Phipunto"
  Bus Creator11/1 -> Bus Creator6/4  "xyzpunto"
  Demux8/3 -> Bus Creator10/3  "Psipunto"
  Demux3/3 -> Bus Creator5/3  "rpunto"
  Demux9/2 -> Bus Creator11/2  "Yepunto"
  Bus Creator7/1 -> Bus Creator6/1  "Vbpunto"
  Bus Creator5/1 -> Bus Creator6/3  "ωpunto"
  Demux9/1 -> Bus Creator11/1  "Xepunto"
  Demux9/3 -> Bus Creator11/3  "Zepunto"
  "PhiThetaPsipunto "/1 -> Demux8/1
  omegapunto/1 -> Demux3/1
  Abb/1 -> Demux4/1
  Bus Creator6/1 -> Xpunto/1

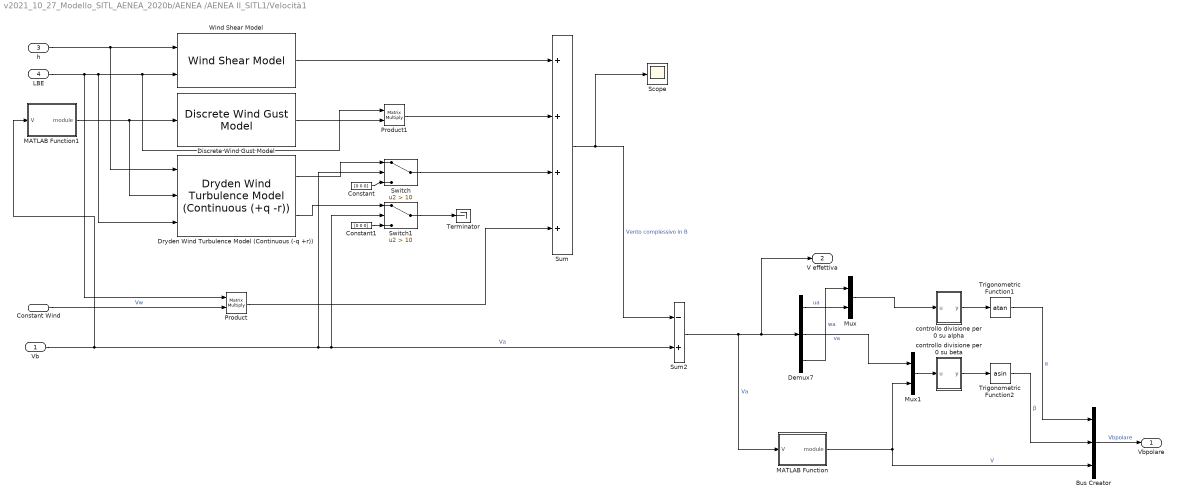
== system v2021_10_27_Modello_SITL_AENEA_2020b/AENEA /AENEA II_SITL1/Velocità1 ==
  Vb : Inport
  Constant Wind : Inport  Port=2
  h : Inport  Port=3
  LBE : Inport  Port=4
  Bus Creator : BusCreator  Inputs=3
  Constant : Constant  Value=[0 0 0]
  Constant1 : Constant  Value=[0 0 0]
  Demux7 : Demux  Outputs=3
  Discrete Wind Gust Model : aerolibwind2/Discrete Wind Gust Model  units=Metric (MKS)  Gx=on  Gy=on  Gz=on  t_0=80  d_m=[120 120 80]  v_m=[0 0 0]
  Dryden Wind Turbulence Model (Continuous (-q +r)) : aerolibwind2/Dryden Wind Turbulence Model  (Continuous (+q -r))  units=Metric (MKS)  spec=MIL-F-8785C  model=Continuous Dryden (-q +r)  W20=0  Wdeg=180  TurbProb=10^-4  L_high=533.4  Wingspan=2.6  ts=0.01  Seed=[23341 23342 23343 23344]  T_on=on
  MATLAB Function : MATLAB Function  TreatAsAtomicUnit=on
  MATLAB Function1 : MATLAB Function  TreatAsAtomicUnit=on
  Mux : Mux  Inputs=2
  Mux1 : Mux  Inputs=2
  Product : Product  Multiplication=Matrix(*)
  Product1 : Product  Multiplication=Matrix(*)
  Scope : Scope
  Sum : Sum  Inputs=4
  Sum2 : Sum  Inputs=-+
  Switch : Switch  Criteria=u2 > Threshold  Threshold=10
  Switch1 : Switch  Criteria=u2 > Threshold  Threshold=10
  Terminator : Terminator
  Trigonometric Function1 : Trigonometry  Operator=atan
  Trigonometric Function2 : Trigonometry  Operator=asin
  Wind Shear Model : aerolibwind2/Wind Shear Model  units=Metric (MKS)  phase=Category C - Terminal Flight Phase  W_20=0  Wdeg=180
  controllo divisione per 0 su alpha : MATLAB Function  TreatAsAtomicUnit=on
  controllo divisione per 0 su beta : MATLAB Function  TreatAsAtomicUnit=on
  Vbpolare : Outport  VectorParamsAs1DForOutWhenUnconnected=off
  "V effettiva " : Outport  Port=2  VectorParamsAs1DForOutWhenUnconnected=off
  wires:
  Bus Creator/1 -> Vbpolare/1  "Vbpolare"
  Trigonometric Function1/1 -> Bus Creator/1  "α"
  MATLAB Function/1(module) -> Mux1/2, Bus Creator/3  "V"
  controllo divisione per 0 su alpha/1(y) -> Trigonometric Function1/1
  controllo divisione per 0 su beta/1(y) -> Trigonometric Function2/1
  Trigonometric Function2/1 -> Bus Creator/2  "β"
  Vb/1 -> MATLAB Function1/1(V), Switch/2, Switch1/2, Sum2/2  "Va"
  Sum2/1 -> "V effettiva "/1, Demux7/1, MATLAB Function/1(V)  "Va"
  Mux/1 -> controllo divisione per 0 su alpha/1(u)
  Demux7/3 -> Mux/1  "wa"
  Demux7/1 -> Mux/2  "ua"
  Mux1/1 -> controllo divisione per 0 su beta/1(u)
  Demux7/2 -> Mux1/1  "va"
  Constant Wind/1 -> Product/2  "Vw"
  h/1 -> Dryden Wind Turbulence Model (Continuous (-q +r))/1, Wind Shear Model/1
  LBE/1 -> Product/1, Dryden Wind Turbulence Model (Continuous (-q +r))/3, Product1/1, Wind Shear Model/2
  Dryden Wind Turbulence Model (Continuous (-q +r))/1 -> Switch/1
  Constant/1 -> Switch/3
  Dryden Wind Turbulence Model (Continuous (-q +r))/2 -> Switch1/1
  Constant1/1 -> Switch1/3
  Wind Shear Model/1 -> Sum/1
  Discrete Wind Gust Model/1 -> Product1/2
  Product1/1 -> Sum/2
  Switch/1 -> Sum/3
  Switch1/1 -> Terminator/1
  Product/1 -> Sum/4
  Sum/1 -> Scope/1, Sum2/1  "Vento complessivo in B"
  MATLAB Function1/1(module) -> Dryden Wind Turbulence Model (Continuous (-q +r))/2, Discrete Wind Gust Model/1

== system v2021_10_27_Modello_SITL_AENEA_2020b/AENEA /AENEA II_SITL1/Weight ==
  LBE : Inport
  Vect_Costanti : Inport  Port=2
  Bus Selector : BusSelector  OutputSignals=Coef_Geometrici.W
  Display1 : Display
  Display3 : Display
  Product3 : Product  Multiplication=Matrix(*)
  "Forzapeso " : Outport  VectorParamsAs1DForOutWhenUnconnected=off
  wires:
  Product3/1 -> "Forzapeso "/1, Display3/1
  LBE/1 -> Product3/1
  Vect_Costanti/1 -> Bus Selector/1
  Bus Selector/1 -> Display1/1, Product3/2  "<W>"

== system v2021_10_27_Modello_SITL_AENEA_2020b/AENEA /toSensors/Calc_GS ==
  In1 : Inport
  Add : Sum
  Demux : Demux  Outputs=3
  Sqrt : Sqrt  SaturateOnIntegerOverflow=on
  Square1 : Math  Operator=square  SignedPower=on  SaturateOnIntegerOverflow=on
  Square2 : Math  Operator=square  SignedPower=on  SaturateOnIntegerOverflow=on
  Terminator : Terminator
  GS : Outport  VectorParamsAs1DForOutWhenUnconnected=off
  wires:
  In1/1 -> Demux/1
  Demux/2 -> Square1/1
  Demux/1 -> Square2/1
  Demux/3 -> Terminator/1
  Square2/1 -> Add/1
  Square1/1 -> Add/2
  Add/1 -> Sqrt/1
  Sqrt/1 -> GS/1

== system v2021_10_27_Modello_SITL_AENEA_2020b/AENEA /toSensors/Calc_heading ==
  In1 : Inport
  Atan2 : Trigonometry  Operator=atan2
  Demux : Demux  Outputs=3
  Terminator : Terminator
  Heading : Outport  VectorParamsAs1DForOutWhenUnconnected=off
  wires:
  In1/1 -> Demux/1
  Demux/3 -> Terminator/1
  Demux/2 -> Atan2/1
  Demux/1 -> Atan2/2
  Atan2/1 -> Heading/1

== system v2021_10_27_Modello_SITL_AENEA_2020b/AENEA /toSensors/To_Lat_Long_MSL ==
  note: Navigation equation
  note: Position derivatives
  V_NED : Inport
  Demux1 : Demux  Outputs=3
      settings: DisplayOption=none
  Demux3 : Demux  Outputs=3
      settings: DisplayOption=none
  Gain : Gain  Gain=-1
  Latitude Bound : Subsystem  mask(Latitude bound){}
      mask help: Bounds the latitude to [-pi/2, pi/2]. When the lower bound is exceeded the latitude is increasing again; when the upper bound is exceeded the latitude is decreasing.
  Longitude Bound : Subsystem  mask(Longitude bound){}
      mask help: Bounds the longitude to [-pi, pi]. When -pi bound is exceeded the longitude wraps back to pi; when the pi bound is exceeded the longitude wraps back to -pi.
  Mux : Mux  Inputs=3
  Mux1 : Mux  Inputs=3
  Position Integrator2 : Integrator  InitialCondition=[latitudineINI longitudineINI HINI]
  Radius at Geocentric Latitude : aerolibasang/Radius at Geocentric Latitude  units=Metric (MKS)  ptype=Earth (WGS84)  F=1/298.257223563  R=6378137
      settings: SourceProductBaseCode=AE
  Sum : Sum  Inputs=|++  InputSameDT=on  SaturateOnIntegerOverflow=on  OutDataTypeStr=Inherit: Same as first input
  Sum1 : Sum  Inputs=|++  InputSameDT=on  SaturateOnIntegerOverflow=on  OutDataTypeStr=Inherit: Same as first input
  Ve/(Rn+h)cos(phi) : Product  Inputs=*//  InputSameDT=on  SaturateOnIntegerOverflow=on  OutDataTypeStr=Inherit: Same as first input
  Vn/(Rm+h) : Product  Inputs=*/  InputSameDT=on  SaturateOnIntegerOverflow=on  OutDataTypeStr=Inherit: Same as first input
  cos(phi) : Trigonometry  Operator=cos
  Position : Outport  VectorParamsAs1DForOutWhenUnconnected=off
  wires:
  Latitude Bound/1(Out) -> cos(phi)/1, Radius at Geocentric Latitude/1, Mux1/1  "lat_optim"
  Longitude Bound/1(Out) -> Mux1/2
  cos(phi)/1 -> Ve/(Rn+h)cos(phi)/3
  Sum1/1 -> Ve/(Rn+h)cos(phi)/2
  Demux3/1 -> Latitude Bound/1(In)
  Ve/(Rn+h)cos(phi)/1 -> Mux/2
  Demux3/2 -> Longitude Bound/1(In)
  Mux1/1 -> Position/1
  Position Integrator2/1 -> Demux3/1
  Demux1/2 -> Ve/(Rn+h)cos(phi)/1
  Mux/1 -> Position Integrator2/1
  Sum/1 -> Vn/(Rm+h)/2
  V_NED/1 -> Demux1/1
  Vn/(Rm+h)/1 -> Mux/1
  Demux3/3 -> Sum/2, Sum1/2, Mux1/3
  Demux1/1 -> Vn/(Rm+h)/1
  Gain/1 -> Mux/3
  Demux1/3 -> Gain/1
  Radius at Geocentric Latitude/1 -> Sum1/1, Sum/1

== system v2021_10_27_Modello_SITL_AENEA_2020b/Ricezione segnali2/Subsystem1/AILERON ==
  In1 : Inport
  Constant : Constant  Value=167
  Gain : Gain  Gain=1/9
  Sum : Sum  Inputs=|+-
  Out1 : Outport  VectorParamsAs1DForOutWhenUnconnected=off
  wires:
  Gain/1 -> Sum/1
  Constant/1 -> Sum/2
  Sum/1 -> Out1/1
  In1/1 -> Gain/1

== system v2021_10_27_Modello_SITL_AENEA_2020b/Ricezione segnali2/Subsystem1/ELEVATOR ==
  In1 : Inport
  Constant : Constant  Value=75175/447
  Gain : Gain  Gain=50/447
  Sum : Sum  Inputs=|+-
  Out1 : Outport  VectorParamsAs1DForOutWhenUnconnected=off
  wires:
  In1/1 -> Gain/1
  Constant/1 -> Sum/2
  Sum/1 -> Out1/1
  Gain/1 -> Sum/1

== system v2021_10_27_Modello_SITL_AENEA_2020b/Ricezione segnali2/Subsystem1/RUDDER ==
  In1 : Inport
  Constant : Constant  Value=75175/447
  Gain : Gain  Gain=50/447
  Sum : Sum  Inputs=|+-
  Out1 : Outport  VectorParamsAs1DForOutWhenUnconnected=off
  wires:
  Gain/1 -> Sum/1
  Constant/1 -> Sum/2
  Sum/1 -> Out1/1
  In1/1 -> Gain/1

== system v2021_10_27_Modello_SITL_AENEA_2020b/Ricezione segnali2/Subsystem1/THROTTLE ==
  In1 : Inport
  Constant : Constant  Value=11/8
  Constant2 : Constant  Value=0
  Gain : Gain  Gain=1/800
  Sum : Sum  Inputs=|+-
  Switch : Switch  Criteria=u2 > Threshold  Threshold=0.003
  Out1 : Outport  VectorParamsAs1DForOutWhenUnconnected=off
  wires:
  In1/1 -> Gain/1
  Constant/1 -> Sum/2
  Gain/1 -> Sum/1
  Switch/1 -> Out1/1
  Sum/1 -> Switch/1, Switch/2
  Constant2/1 -> Switch/3

== system v2021_10_27_Modello_SITL_AENEA_2020b/AENEA /AENEA II_SITL1/Forze aerodinamiche/Forze assi vento//q ==
  Vect_Comandi : Inport
  Vect_Costanti : Inport  Port=2
  "Vbpolare " : Inport  Port=3
  ωb : Inport  Port=4
  Bus Creator : BusCreator  Inputs=3
  Bus Selector : BusSelector  OutputSignals=deltaE
  Bus Selector1 : BusSelector  OutputSignals=p,r,q
  Display : Display
  Gain4 : Gain  Gain=-1
  Gain5 : Gain  Gain=-1
  Scope : Scope
  Subsystem : Subsystem
  Subsystem1 : Subsystem
  Subsystem2 : Subsystem
  FA_W/q : Outport  VectorParamsAs1DForOutWhenUnconnected=off
  CL : Outport  Port=2  VectorParamsAs1DForOutWhenUnconnected=off
  wires:
  Bus Selector/1 -> Subsystem2/2(deltaE)  "<deltaE>"
  Subsystem/1(CD) -> Display/1, Scope/1, Gain4/1
  Subsystem2/1(CL) -> CL/1, Gain5/1
  Vect_Costanti/1 -> Subsystem2/3(Vect_Costanti), Subsystem1/3(Vect_Costanti), Subsystem/1(Vect_Costanti)
  Vect_Comandi/1 -> Subsystem1/4(Vect_Comandi), Bus Selector/1
  "Vbpolare "/1 -> Subsystem1/5("Vbpolare "), Subsystem2/4("Vbpolare "), Subsystem/2("Vbpolare ")
  ωb/1 -> Bus Selector1/1
  Bus Selector1/1 -> Subsystem1/1(p)  "<p>"
  Bus Selector1/3 -> Subsystem2/1(q)  "<q>"
  Bus Selector1/2 -> Subsystem1/2(r)  "<r>"
  Bus Creator/1 -> FA_W/q/1
  Gain5/1 -> Bus Creator/3  "CL"
  Subsystem1/1("CY ") -> Bus Creator/2  "CY"
  Gain4/1 -> Bus Creator/1  "CD"

== system v2021_10_27_Modello_SITL_AENEA_2020b/AENEA /AENEA II_SITL1/Forze aerodinamiche/Momenti //press din ==
  Vect_Comandi : Inport
  Vect_Costanti : Inport  Port=2
  "Vbpolare " : Inport  Port=3
  ωb : Inport  Port=4
  Bus Creator : BusCreator  Inputs=3
  Bus Selector : BusSelector  OutputSignals=Coef_Geometrici.S*b,Coef_Geometrici.S*cbar
  Product : Product
  Product1 : Product
  Product3 : Product
  Subsystem3 : Subsystem
  Subsystem4 : Subsystem
  Subsystem5 : Subsystem
  MA_B/q : Outport  VectorParamsAs1DForOutWhenUnconnected=off
  wires:
  Subsystem5/1(Cn) -> Product3/2
  Subsystem4/1(Cm) -> Product1/2
  Subsystem3/1(Cl) -> Product/2
  Vect_Costanti/1 -> Bus Selector/1, Subsystem3/1(Vect_Costanti), Subsystem5/1(Vect_Costanti), Subsystem4/1(Vect_Costanti)
  Vect_Comandi/1 -> Subsystem4/2(Vect_Comandi), Subsystem3/2(Vect_Comandi), Subsystem5/2(Vect_Comandi)
  "Vbpolare "/1 -> Subsystem5/3("Vbpolare "), Subsystem4/3("Vbpolare "), Subsystem3/3("Vbpolare ")
  ωb/1 -> Subsystem5/4(ωb), Subsystem4/4(ωb), Subsystem3/4(ωb)
  Bus Selector/1 -> Product3/1, Product/1  "<S*b>"
  Bus Selector/2 -> Product1/1  "<S*cbar>"
  Bus Creator/1 -> MA_B/q/1
  Product/1 -> Bus Creator/1  "Cl"
  Product1/1 -> Bus Creator/2  "Cm"
  Product3/1 -> Bus Creator/3  "Cn"

== system v2021_10_27_Modello_SITL_AENEA_2020b/AENEA /AENEA II_SITL1/Propulsione1/LUT ELICA  ==
  J : Inport
  RPM : Inport  Port=2
  Constant : Constant  Value=matricepolinomi  VectorParams1D=off
  MATLAB Function : MATLAB Function  TreatAsAtomicUnit=on
  Ct : Outport  VectorParamsAs1DForOutWhenUnconnected=off
  Cp : Outport  Port=2  VectorParamsAs1DForOutWhenUnconnected=off
  wires:
  MATLAB Function/2(Cp) -> Cp/1  "Cp"
  J/1 -> MATLAB Function/1(J)
  Constant/1 -> MATLAB Function/3(matricepolinomi)
  MATLAB Function/1(Ct) -> Ct/1  "Ct"
  RPM/1 -> MATLAB Function/2(RPM)

== system v2021_10_27_Modello_SITL_AENEA_2020b/AENEA /AENEA II_SITL1/Propulsione1/LUT ELICA 1 ==
  J : Inport
  RPM : Inport  Port=2
  2-D Lookup Table : Lookup_n-D  BreakpointsForDimension1=J_vec  BreakpointsForDimension2=RPM_vec(2:end)  Table=Ct(2:end,2:end)  InternalRulePriority=Speed  RndMeth=Simplest  InputSameDT=on
      settings: InputPortMap=u0,u1
  2-D Lookup Table1 : Lookup_n-D  BreakpointsForDimension1=J_vec  BreakpointsForDimension2=RPM_vec(2:end)  Table=Cp(2:end,2:end)  InternalRulePriority=Speed  RndMeth=Simplest  InputSameDT=on
      settings: InputPortMap=u0,u1
  Ct : Outport  VectorParamsAs1DForOutWhenUnconnected=off
  Cp : Outport  Port=2  VectorParamsAs1DForOutWhenUnconnected=off
  wires:
  RPM/1 -> 2-D Lookup Table/2, 2-D Lookup Table1/2
  J/1 -> 2-D Lookup Table1/1, 2-D Lookup Table/1
  2-D Lookup Table1/1 -> Cp/1
  2-D Lookup Table/1 -> Ct/1

== system v2021_10_27_Modello_SITL_AENEA_2020b/AENEA /AENEA II_SITL1/Propulsione1/Subsystem1 ==
  T : Inport
  P : Inport  Port=2
  RPS : Inport  Port=3
  V_cost : Inport  Port=4
  Bus Selector : BusSelector  OutputSignals=Coef_Propulsivi.Zeng
  Constant : Constant  Value=0
  Constant1 : Constant  Value=0
  Divide : Product  Inputs=*/
  Divide1 : Product  Inputs=**
  Gain : Gain  Gain=2*pi
  Gain1 : Gain  Gain=-1
  Mux : Mux  Inputs=3
  Mux1 : Mux  Inputs=3
  Fthrust : Outport  VectorParamsAs1DForOutWhenUnconnected=off
  "Mthrust " : Outport  Port=2  VectorParamsAs1DForOutWhenUnconnected=off
  wires:
  T/1 -> Divide1/2, Mux/1
  Constant/1 -> Mux/2, Mux/3
  Mux/1 -> Fthrust/1
  RPS/1 -> Gain/1
  P/1 -> Divide/1
  Gain/1 -> Divide/2
  Gain1/1 -> Mux1/1
  Divide/1 -> Gain1/1
  Divide1/1 -> Mux1/2
  Constant1/1 -> Mux1/3
  Mux1/1 -> "Mthrust "/1
  V_cost/1 -> Bus Selector/1
  Bus Selector/1 -> Divide1/1  "<Zeng>"

== system v2021_10_27_Modello_SITL_AENEA_2020b/AENEA /AENEA II_SITL1/Propulsione1/Subsystem2 ==
  T : Inport
  P : Inport  Port=2
  RPS : Inport  Port=3
  Constant : Constant  Value=0
  Constant1 : Constant  Value=0
  Divide : Product  Inputs=*/
  Gain : Gain  Gain=2*pi
  Gain1 : Gain  Gain=-1
  Mux : Mux  Inputs=3
  Mux1 : Mux  Inputs=3
  "xprop " : Gain  Gain=-0.15
  Fthrust : Outport  VectorParamsAs1DForOutWhenUnconnected=off
  "Mthrust " : Outport  Port=2  VectorParamsAs1DForOutWhenUnconnected=off
  wires:
  T/1 -> "xprop "/1, Mux/1
  Constant/1 -> Mux/2, Mux/3
  Mux/1 -> Fthrust/1
  RPS/1 -> Gain/1
  P/1 -> Divide/1
  Gain/1 -> Divide/2
  Gain1/1 -> Mux1/1
  Divide/1 -> Gain1/1
  "xprop "/1 -> Mux1/2
  Constant1/1 -> Mux1/3
  Mux1/1 -> "Mthrust "/1

== system v2021_10_27_Modello_SITL_AENEA_2020b/AENEA /toSensors/To_Lat_Long_MSL/Latitude Bound ==
  In : Inport
  2pi : Constant  Value=2*pi
  ChSign : Gain  Gain=-1  SaturateOnIntegerOverflow=on  OutDataTypeStr=Inherit: Same as input  ParamDataTypeStr=Inherit: Same as input
  Math Function : Math  Operator=mod  SignedPower=on  SaturateOnIntegerOverflow=on
  Math Function1 : Math  Operator=mod  SignedPower=on  SaturateOnIntegerOverflow=on
  Sum1 : Sum  Inputs=|+-  InputSameDT=on  SaturateOnIntegerOverflow=on  OutDataTypeStr=Inherit: Same as first input
  Sum2 : Sum  Inputs=|++  InputSameDT=on  SaturateOnIntegerOverflow=on  OutDataTypeStr=Inherit: Same as first input
  Switch : Switch  Threshold=pi  SaturateOnIntegerOverflow=on  InputSameDT=on
  pi : Constant  Value=pi
  pi/2 : Constant  Value=pi/2
  Out : Outport  VectorParamsAs1DForOutWhenUnconnected=off
  wires:
  pi/1 -> Math Function/2
  Math Function/1 -> Sum1/1
  pi/2/1 -> Sum1/2, Sum2/2
  Sum1/1 -> ChSign/1, Switch/3
  Math Function1/1 -> Switch/2
  Switch/1 -> Out/1
  In/1 -> Sum2/1
  Sum2/1 -> Math Function/1, Math Function1/1
  ChSign/1 -> Switch/1
  2pi/1 -> Math Function1/2

== system v2021_10_27_Modello_SITL_AENEA_2020b/AENEA /toSensors/To_Lat_Long_MSL/Longitude Bound ==
  In : Inport
  2pi : Constant  Value=2*pi
  Math Function : Math  Operator=mod  SignedPower=on  SaturateOnIntegerOverflow=on
  Sum1 : Sum  Inputs=|+-  InputSameDT=on  SaturateOnIntegerOverflow=on  OutDataTypeStr=Inherit: Same as first input
  Sum2 : Sum  Inputs=|++  InputSameDT=on  SaturateOnIntegerOverflow=on  OutDataTypeStr=Inherit: Same as first input
  pi : Constant  Value=pi
  Out : Outport  VectorParamsAs1DForOutWhenUnconnected=off
  wires:
  Sum1/1 -> Out/1
  pi/1 -> Sum1/2, Sum2/2
  Sum2/1 -> Math Function/1
  In/1 -> Sum2/1
  2pi/1 -> Math Function/2
  Math Function/1 -> Sum1/1
